simulink model "Vehicle_Model_999_Modular_roll_gradient"  (R2025b)
settings: Solver=ode23tb  StartTime=0.0  StopTime=30  MaxStep=0.001  RelTol=1e-3
values from neighbouring files (symbols this model uses):
  m = Par.m    [LapSim_Endurance_final_ts_v2.m]    (also in New_LapSim_final_ts.m = Par.Mass)
undefined symbols (not defined in the file or in its folder): Battery, Brake_Val, ctrl_Brake, ctrl_s, ctrl_Steer, ctrl_Throttle, ctrl_Velocity, HP, init_r, init_vx, init_vy, Ki_data, Kp_data, Motor, Par, steer_input, Steer_Val, sus_par, Throttle_Val, TireData, V_ref, vx_breakpoints
libraries: simulink x8, autolibshared x3, simulink_extras x2, BatteryEstimators x1
(part 3 of 3)

== matlab function Vehicle_Model_999_Modular_roll_gradient/E-powertrain/Motor/Motor with Field Weakening ==
  data: kt input; rpm_4x1 input; Torque_Nm_vec output; throttle_scalar input; v_dc_bus input; Motor parameter; I_dc_total output size=[1]; P_total_sum output size=[1]
function [Torque_Nm_vec, I_dc_total,P_total_sum] = fcn(kt, rpm_4x1, throttle_scalar, v_dc_bus, Motor)
    % Inputs:
    %   rpm_4x1         : [FL; FR; RL; RR] wheel speeds in RPM
    %   throttle_scalar : Driver input (0 to 1)
    %   v_dc_bus        : Battery voltage (V)
    %   Motor           : Struct containing constants
    
    % --- 1. Distribute Inputs ---
    % We apply the same throttle to both motors for now.
    % We extract the Rear-Left (index 3) and Rear-Right (index 4) speeds.
    rpm_targets = [rpm_4x1(3); rpm_4x1(4)]; 
    throttle_vec = [throttle_scalar; throttle_scalar];
    psi_m = kt / (1.5 * Motor.p * sqrt(2)); 

    % Initialize storage
    Torque_Nm_vec = zeros(2, 1); % [T_RL; T_RR]
    P_elec_vec = zeros(2, 1);
    
    for i = 1:2
        % --- 2. Redline & Mechanical Limit Check ---
        if abs(rpm_targets(i)) >= Motor.n_max
            continue; % Torque and Power remain 0
        end

        % --- 3. Electrical Conversions ---
        omega_m = rpm_targets(i) * (2*pi/60);
        omega_e = max(abs(omega_m * Motor.p), 0.1); 
        V_max_phase = v_dc_bus / sqrt(3);
        I_cmd_peak = Motor.I_max_rms * sqrt(2) * throttle_vec(i);

        % --- 4. Region Selection: MTPA vs Field Weakening ---
        V_req_mtpa = omega_e * sqrt((Motor.L * I_cmd_peak)^2 + psi_m^2);
        
        if V_req_mtpa <= V_max_phase
            id = 0;
            iq = I_cmd_peak;
        else
            % Field Weakening logic for Fischer Motor
            a = Motor.L^2;
            b = 2 * Motor.L * psi_m;
            c = Motor.psi_m^2 + (Motor.L * I_cmd_peak)^2 - (V_max_phase / omega_e)^2;
            
            id = (-b + sqrt(max(0, b^2 - 4 * a * c))) / (2 * a);
            id = max(min(id, 0), -I_cmd_peak); 
            iq = sqrt(max(0, I_cmd_peak^2 - id^2));
        end

        % --- 5. Torque and Power Calculation ---
        T_gen = 1.5 * Motor.p * psi_m * iq;
        Torque_Nm_vec(i) = min(T_gen, Motor.T_peak_limit);

        % P_elec = P_mechanical + P_copper_losses
        P_mech = abs(Torque_Nm_vec(i) * omega_m);
        P_copper = 3 * 0.126 * (I_cmd_peak / sqrt(2))^2;
        P_elec_vec(i) = P_mech + P_copper;
    end

    % --- 6. Battery Summation ---
    P_total_sum = sum(P_elec_vec);
    if v_dc_bus > 20
        % Calculate total current draw for the Molicel P45B pack
        I_dc_total = P_total_sum / (0.95 * v_dc_bus);

    else
        I_dc_total = 0;
    end
end

== matlab function Vehicle_Model_999_Modular_roll_gradient/Vehicle dynamics/Suspension/MATLAB Function1 ==
  data: vel input; aerodynamic_downforce output; aero_par parameter
function aerodynamic_downforce = fcn(vel,aero_par)

rho = aero_par.rho;
cd = aero_par.Cd;
A = aero_par.Area;

aerodynamic_downforce = 0.5*rho*cd*A*vel^2;

== matlab function Vehicle_Model_999_Modular_roll_gradient/Vehicle dynamics/Suspension/Roll and pitch angle calculations/Pitch_angle_calcualtions ==
  data: z_wheel input size=[4 1]; Pitch_angle output; Par parameter
function Pitch_angle = fcn(z_wheel,Par)

WB = Par.WB;

% Avg disp calculation per axle 
z_avg_f = (z_wheel(1) + z_wheel(2))/2;
z_avg_r = (z_wheel(3) + z_wheel(4))/2;

Pitch_angle = (z_avg_r- z_avg_f)/WB;

== matlab function Vehicle_Model_999_Modular_roll_gradient/Vehicle dynamics/Suspension/Roll and pitch angle calculations/Roll_angle_calulations ==
  data: z_wheel input size=[4 1]; Roll_angle output; Par parameter
function Roll_angle = fcn(z_wheel,Par)

TW = Par.TW;

% Avg disp calculation per track
z_avg_l = (z_wheel(1) + z_wheel(3))/2;
z_avg_r = (z_wheel(2) + z_wheel(4))/2;

Roll_angle = (z_avg_l - z_avg_r)/TW;

== matlab function Vehicle_Model_999_Modular_roll_gradient/Vehicle dynamics/Suspension/MATLAB Function2 ==
  data: Z_dyn input; Camber output; Camber_gain output; HP parameter; sus_par parameter
function [Camber, Camber_gain] = DynamicCamber_FromHP_Zmeters(Z_dyn, HP, sus_par)
%#codegen
% Z_dyn : dynamic wheel vertical displacement from static ride height (meters, + = bump)
% Output Camber [4x1] radians (dynamic absolute camber)

% 1. Configured static camber
static_camber_4x1 = sus_par.Camber_static .* ones(4,1);

% 2. Dynamic displacements in mm (FL, FR, RL, RR)
zw = Z_dyn .* [sus_par.Motion_ratio_f; sus_par.Motion_ratio_f; ...
               sus_par.Motion_ratio_r; sus_par.Motion_ratio_r] .* 1000;

% 3. Extract and Vectorize Hardpoints (Applying side mirroring directly)
% Inner Pivots (Y and Z) - Average of F and R legs to establish the inner pivot axis
UiY = [ (HP.Front.UCA_F(2) + HP.Front.UCA_R(2))*0.5;
       -(HP.Front.UCA_F(2) + HP.Front.UCA_R(2))*0.5;
        (HP.Rear.UCA_F(2)  + HP.Rear.UCA_R(2))*0.5;
       -(HP.Rear.UCA_F(2)  + HP.Rear.UCA_R(2))*0.5 ];

UiZ = [ (HP.Front.UCA_F(3) + HP.Front.UCA_R(3))*0.5;
        (HP.Front.UCA_F(3) + HP.Front.UCA_R(3))*0.5;
        (HP.Rear.UCA_F(3)  + HP.Rear.UCA_R(3))*0.5;
        (HP.Rear.UCA_F(3)  + HP.Rear.UCA_R(3))*0.5 ];

LiY = [ (HP.Front.LCA_F(2) + HP.Front.LCA_R(2))*0.5;
       -(HP.Front.LCA_F(2) + HP.Front.LCA_R(2))*0.5;
        (HP.Rear.LCA_F(2)  + HP.Rear.LCA_R(2))*0.5;
       -(HP.Rear.LCA_F(2)  + HP.Rear.LCA_R(2))*0.5 ];

LiZ = [ (HP.Front.LCA_F(3) + HP.Front.LCA_R(3))*0.5;
        (HP.Front.LCA_F(3) + HP.Front.LCA_R(3))*0.5;
        (HP.Rear.LCA_F(3)  + HP.Rear.LCA_R(3))*0.5;
        (HP.Rear.LCA_F(3)  + HP.Rear.LCA_R(3))*0.5 ];

% Outer Pivots (Y and Z base static values)
UO_Y = [HP.Front.UCA_O(2); -HP.Front.UCA_O(2); HP.Rear.UCA_O(2); -HP.Rear.UCA_O(2)];
LO_Y = [HP.Front.LCA_O(2); -HP.Front.LCA_O(2); HP.Rear.LCA_O(2); -HP.Rear.LCA_O(2)];
TCP_Y = [HP.Front.TCP(2);  -HP.Front.TCP(2);  HP.Rear.TCP(2);  -HP.Rear.TCP(2)];

UO_Z_base  = [HP.Front.UCA_O(3); HP.Front.UCA_O(3); HP.Rear.UCA_O(3); HP.Rear.UCA_O(3)];
LO_Z_base  = [HP.Front.LCA_O(3); HP.Front.LCA_O(3); HP.Rear.LCA_O(3); HP.Rear.LCA_O(3)];
TCP_Z_base = [HP.Front.TCP(3);   HP.Front.TCP(3);   HP.Rear.TCP(3);   HP.Rear.TCP(3)];

% 4. Compute Kinematics Vectorized (All 4 corners at once)
% Dynamic geometry
Camber_d = compute_corner_kinematics(zw, UiY, UiZ, LiY, LiZ, UO_Y, LO_Y, TCP_Y, UO_Z_base, LO_Z_base, TCP_Z_base);

% Static geometry (0 mm travel)
Camber_s_raw = compute_corner_kinematics([0;0;0;0], UiY, UiZ, LiY, LiZ, UO_Y, LO_Y, TCP_Y, UO_Z_base, LO_Z_base, TCP_Z_base);
Camber_s = abs(Camber_s_raw); % Mirroring your original solveCorner_theta logic

% 5. Calculate Deltas (Preserving your exact original quadrant/sign logic)
Camber_delta = [
    -Camber_s(1) + Camber_d(1);
    -Camber_d(2) - Camber_s(2);
     Camber_d(3) - Camber_s(3);
    -Camber_d(4) - Camber_s(4)
];

% 6. Final Outputs
Camber = Camber_delta + static_camber_4x1;
Camber_gain = Camber_d;
static_camber_visualisation = Camber_s;

end

%% High-Performance Vectorized Helper Function
function Camber_rad = compute_corner_kinematics(zw, UiY, UiZ, LiY, LiZ, UO_Y, LO_Y, TCP_Y, UO_Z_base, LO_Z_base, TCP_Z_base)
    % Apply vertical travel
    UO_Z  = UO_Z_base + zw;
    LO_Z  = LO_Z_base + zw;
    TCP_Z = TCP_Z_base + zw;

    % Slopes of upper & lower arms
    dYU = UO_Y - UiY;
    dYL = LO_Y - LiY;

    % Singularity protection (Replaces previous 0*sign(0) bug)
    dYU = protect_zero(dYU, 1e-6);
    dYL = protect_zero(dYL, 1e-6);

    mU = (UO_Z - UiZ) ./ dYU;
    mL = (LO_Z - LiZ) ./ dYL;

    cU = UiZ - mU .* UiY;
    cL = LiZ - mL .* LiY;

    % Instant Center (IC) Calculation
    den = mU - mL;
    den = protect_zero(den, 1e-6);

    ICy = (cL - cU) ./ den;
    ICz = mU .* ICy + cU;

    % Camber from IC to Contact Patch
    dY = ICy - TCP_Y;
    dZ = ICz - TCP_Z;
    dZ = protect_zero(dZ, 1e-6);

    Camber_rad = -atan(dY ./ dZ);
end

%% Singularity Protection Helper (Coder Safe)
function out = protect_zero(val, tol)
    out = val;
    for i = 1:4
        if abs(out(i)) < tol
            s = sign(out(i));
            if s == 0
                s = 1;
            end
            out(i) = s * tol;
        end
    end
end

== matlab function Vehicle_Model_999_Modular_roll_gradient/Vehicle dynamics/Fx, Fy calculations/Tyre_relaxation/MATLAB Function ==
  data: Fx_ss input; Fx_dot output; Fx_act input; Vx input
function Fx_dot = fcn(Fx_ss, Fx_act, Vx)
    % Fx_ss: Force from Magic Formula block
    % Fx_act: The current integrated force
    % Vx: Longitudinal velocity
    sigma_x = 0.1;
    % Use a small epsilon to avoid division by zero at standstill
    Vx_mod = max(abs(Vx), 0.05); 
    
    % The differential equation
    Fx_dot = (Vx_mod / sigma_x).* (Fx_ss - Fx_act);
end

== matlab function Vehicle_Model_999_Modular_roll_gradient/Vehicle dynamics/Fx, Fy calculations/Visualise_Fy_B/MATLAB Function ==
  data: Fy_tire input; Fy_B_fl output; Fy_B_fr output; Fy_B_rl output; Fy_B_rr output
function [Fy_B_fl,Fy_B_fr,Fy_B_rl,Fy_B_rr]  = fcn(Fy_tire)

Fy_B_fl = Fy_tire(1);

Fy_B_fr = Fy_tire(2);

Fy_B_rl = Fy_tire(3);

Fy_B_rr = Fy_tire(4);

end

== matlab function Vehicle_Model_999_Modular_roll_gradient/Drivetrain/MATLAB Function ==
  data: T_fl output; T_fr output
function [T_fl,T_fr] = fcn()

T_fl = 0;
T_fr = 0;

== matlab function Vehicle_Model_999_Modular_roll_gradient/E-powertrain/Motor/rpm selection for third wheel ==
  data: u input; y output
function y = fcn(u)

y = u(3);

== matlab function Vehicle_Model_999_Modular_roll_gradient/Vehicle dynamics/Fx, Fy calculations/Slip_angle_calculation/Slip Angles ==
  data: Longitudinal_vel input; slip_angles output; Lateral_vel input; yawrate input; Steer_FL input; Steer_FR input; Par parameter
function slip_angles = fcn(Longitudinal_vel, Lateral_vel, yawrate, Steer_FL, Steer_FR, Par)
%#codegen

    % 1. Geometry Setup
    L = Par.WB;
    T = Par.TW;
    
    % Distance from CG to Axles
    a = L * Par.WD_r;     
    b = L - a;             
    half_T = T / 2;

    % 2. Calculate Velocity Components at Each Corner
    % Kinematic transformation from CG to Hubs
    % Front Left (1)
        Vx_FL = Longitudinal_vel - yawrate * half_T;
        Vy_FL = Lateral_vel + yawrate * a;
    
    % Front Right (2)
        Vx_FR = Longitudinal_vel + yawrate * half_T;
        Vy_FR = Lateral_vel + yawrate * a;
    
    % Rear Left (3)
        Vx_RL = Longitudinal_vel - yawrate * half_T;
        Vy_RL = Lateral_vel - yawrate * b;
    
    % Rear Right (4)
        Vx_RR = Longitudinal_vel + yawrate * half_T;
        Vy_RR = Lateral_vel - yawrate * b;

    % 3. Calculate Velocity Angles (Theta_V)

        Theta_FL = atan2(Vy_FL, max(Vx_FL,0.001)); 
        Theta_FR = atan2(Vy_FR, max(Vx_FR,0.001));
        Theta_RL = atan2(Vy_RL, max(Vx_RL,0.001));
        Theta_RR = atan2(Vy_RR, max(Vx_RR,0.001));
    
    % 4. Construct Steering Vector (Delta)
    % Rears are assumed fixed (0 steering)
        Delta = [Steer_FL; Steer_FR; 0; 0];
    
    % Vector of Velocity Angles
        Theta_V = [Theta_FL; Theta_FR; Theta_RL; Theta_RR];

    % 5. Final Calculation
    % Alpha = Delta - Theta_V
        slip_angles = Delta - Theta_V ;
end

== matlab function Vehicle_Model_999_Modular_roll_gradient/Vehicle dynamics/Fx, Fy calculations/Slip_ratio_calculation/slip ratios ==
  data: Vx input; Vy input; slip_ratios output; yawrate input; Omega input; Steer_FL input; Steer_FR input; Par parameter
function slip_ratios = fcn(Vx,Vy, yawrate, Omega,Steer_FL,Steer_FR, Par)
%#codegen


    % 1. Constants
    T = Par.TW;
    Re = Par.R0;
    half_T = T / 2;
    a= Par.Lf;
    b=Par.Lr;
    r = yawrate;
    % 2 Yaw Rate Correction (Kinematics)
    
    Vx_FL = Vx - yawrate * half_T;  % Left
    Vx_FR = Vx + yawrate * half_T;  % Right
    Vx_RL = Vx - yawrate * half_T;
    Vx_RR = Vx + yawrate * half_T;
    
    Vx_vec = [Vx_FL; Vx_FR; Vx_RL; Vx_RR];
    
    Vy_FL = Vy + r * a;
    Vy_FR = Vy+ r * a;
    Vy_RL = Vy- r * b;
    Vy_RR = Vy- r * b;

    Vy_vec = [Vy_FL; Vy_FR; Vy_RL; Vy_RR];
    Delta = [Steer_FL;Steer_FR;0;0];
    % 3. Slip Angle Correction (Projection)
 
    V_road_plane = Vx_vec .* cos(Delta) + Vy_vec .* sin(Delta);

    % 4. Calculate Wheel Linear Speed
    V_wheel = Omega .* Re;

    % 5. Calculate Slip Ratio
    V_safe_threshold = 0.1; 
    V_ref = max(abs(V_road_plane), V_safe_threshold);
    
    slip_ratios_raw = (V_wheel - V_road_plane) ./ V_ref;
    slip_ratios = slip_ratios_raw;
    % slip_ratios = min(max(slip_ratios_raw,-1),1);
end

== matlab function Vehicle_Model_999_Modular_roll_gradient/Vehicle dynamics/Steering/Steering Kinematics/Steering Kinematics ==
  data: Steer_Input input; Ackermann_Pct input; Steer_FL output; Steer_FR output; Par parameter
function [Steer_FL, Steer_FR] = fcn(Steer_Input, Ackermann_Pct, Par)
%#codegen

    % 1. Constants
    L = Par.WB;      % Wheelbase
    half_T = Par.TW / 2; % Half Track Width

    % 2. Safety Clamp (Prevent tan(90) singularity)
    delta = min(max(Steer_Input, -1.5), 1.5); 
    
    % 3. Calculate "Pure Ackermann" Angles
    % Ideally, inner wheel turns sharper than outer wheel.
    tan_d = tan(delta);
    
    % FL (Left): Denom depends on sign of turn.
    % If turning Left (+), Denom shrinks (Sharper).
    FL_Ack = atan( (L * tan_d) / (L - half_T * tan_d) );
    
    % FR (Right): 
    % If turning Left (+), Denom grows (Shallower).
    FR_Ack = atan( (L * tan_d) / (L + half_T * tan_d) );
    
    % 4. Calculate "Parallel" Angles
    % Both wheels exactly match the center input
    FL_Par = delta;
    FR_Par = delta;
    
    % 5. Linear Blend based on Percentage
    % Formula: Final = Parallel + (Ackermann - Parallel) * Percent
    Steer_FL = FL_Par + (FL_Ack - FL_Par) * Ackermann_Pct;
    Steer_FR = FR_Par + (FR_Ack - FR_Par) * Ackermann_Pct;

end

== matlab function Vehicle_Model_999_Modular_roll_gradient/Vehicle dynamics/Fx, Fy calculations/Simplified Tire Model ==
  data: Fz input; Fx output size=4; slip_ratios input; slip_angles input; camber_angles input; Fy output size=4; Self_aligning_torque output size=4; Mu_x output size=4; Mu_y output size=4; TireData parameter; Par parameter; sus_par parameter; Dy output size=[4 1]
function [Fx, Fy, Self_aligning_torque, Mu_x, Mu_y, Dy] = fcn(Fz, slip_ratios, slip_angles, camber_angles, TireData, Par, sus_par)
%#codegen
% =========================================================================
%  VECTORIZED MAGIC FORMULA 5.2 (4-WHEEL)
% =========================================================================

    % 0. Enforce Column Vectors (Crash Protection)
    Fz = Fz(:);
    slip_ratios = slip_ratios(:);
    slip_angles = slip_angles(:);
    camber_angles = camber_angles(:);

    % 1. EXTRACT PARAMETERS (Scalars)
    p = TireData;
    s = TireData.Scales;
    Fz0 = p.FNOMIN;
    R0  = p.R0;
    par = Par;
    
    % 2. INPUT SAFETY & NORMALIZATION
    % Clamp negative loads to 0 (Tires can't pull ground)
    Fz_safe = max(Fz, 0); 
    
    % Avoid division by zero for Mu calculations later
    Fz_denom = max(Fz_safe, 1.0); 
    
    % Normalized Load (dfz) - Vectorized
    dfz = (Fz_safe - Fz0) ./ Fz0;
    
    % ---------------------------------------------------------------------
    % A. LONGITUDINAL FORCE (Fx) - VECTORIZED
    % ---------------------------------------------------------------------
    Cx = p.PCX1 * s.LCX;
    
    % Friction Coeff Mu_x
    mu_x_base = (p.PDX1 + p.PDX2 .* dfz) .* (1 - p.PDX3 .* camber_angles.^2) .* s.LMUX;
    Dx = mu_x_base .* Fz_safe;
    
    % Stiffness Kx
    Kx = Fz_safe .* (p.PKX1 + p.PKX2 .* dfz) .* exp(p.PKX3 .* dfz) .* s.LKX;
    
    % Stiffness Factor Bx
    Bx = Kx ./ (Cx .* Dx + 1e-6); 
    
    % Shifts (Horizontal & Vertical)
    Shx = (p.PHX1 + p.PHX2 .* dfz) .* s.LHX;
    Svx = Fz_safe .* (p.PVX1 + p.PVX2 .* dfz) .* s.LVX;
    
    % Composite Slip
    k_s = slip_ratios + Shx;
    
    % Curvature Ex (Sign Dependent)
    Ex = (p.PEX1 + p.PEX2 .* dfz + p.PEX3 .* dfz.^2) .* (1 - p.PEX4 .* sign(k_s)) .* s.LEX;
    Ex(Ex > 1) = 1; % Clamp
    
    % Calculation
    Bx_k = Bx .* k_s;
    Fx = Dx .* sin(Cx .* atan(Bx_k - Ex .* (Bx_k - atan(Bx_k)))) + Svx;
    
    % ---------------------------------------------------------------------
    % B. LATERAL FORCE (Fy) - VECTORIZED
    % ---------------------------------------------------------------------
    Cy = p.PCY1 * s.LCY;
    
    % Friction Coeff Mu_y
    mu_y_base = (p.PDY1 + p.PDY2 .* dfz) .* (1 - p.PDY3 .* camber_angles.^2) .* s.LMUY;
    Dy = mu_y_base .* Fz_safe;
    
    % Cornering Stiffness Ky (Trig Form)
    Ky = p.PKY1 .* Fz0 .* sin(2 .* atan(Fz_safe ./ (p.PKY2 .* Fz0))) .* (1 - p.PKY3 .* abs(camber_angles)) .* s.LKY;
    
    % Poly fallback check (if PKY2 implies poly form)
    if (Ky(1) < 1)
        Ky = Fz_safe .* (p.PKY1 + p.PKY2 .* dfz) .* s.LKY;
    end
    
    By = Ky ./ (Cy .* Dy + 1e-6);
    
    % Shifts 
    Shy = (p.PHY1 + p.PHY2 .* dfz) .* s.LHY;
    Svy = Fz_safe .* (p.PVY1 + p.PVY2 .* dfz) .* s.LVY;
    
    % FIXED: Removed the 0* debug multiplier
    a_s = slip_angles + Shy;
    
    % Curvature Ey (Sign Dependent)
    Ey = (p.PEY1 + p.PEY2 .* dfz) .* (1 - (p.PEY3 + p.PEY4 .* camber_angles) .* sign(a_s)) .* s.LEY;
    Ey(Ey > 1) = 1;
    
    % Calculation
    By_a = By .* a_s;
    % FIXED: Removed the 0* debug multiplier
    Fy = -(Dy .* sin(Cy .* atan(By_a - Ey .* (By_a - atan(By_a)))) + Svy);
    
    % ---------------------------------------------------------------------
    % C. SELF-ALIGNING TORQUE (Mz) - VECTORIZED
    % ---------------------------------------------------------------------
    % Peak Trail Dt
    Dt = (p.QDZ1 + p.QDZ2 .* dfz) .* (1 - p.QDZ3 .* abs(camber_angles)) .* R0 .* s.LTR;
    
    % Trail Slope Bt
    Bt = (p.QBZ1 + p.QBZ2 .* dfz + p.QBZ3 .* dfz.^2) .* (1 + p.QBZ4 .* abs(camber_angles)) .* (s.LKY / s.LMUY);
    
    Ct = p.QCZ1; % Scalar
    Et = (p.QEZ1 + p.QEZ2 .* dfz + p.QEZ3 .* dfz.^2);
    
    % Trail 't' Calculation(Pneumatic trail)
    Bt_a = Bt .* a_s;
    alpha_t = Bt_a - Et .* (Bt_a - atan(Bt_a));
    t = Dt .* cos(Ct .* atan(alpha_t)) .* cos(a_s);
    
    % Trail 'tm' Calculation(mechanical trail)
    tm = par.R0 .* tan(sus_par.Caster_static);
    
    % Residual Mzr
    Dr = Fz_safe .* R0 .* (p.QDZ6 + p.QDZ7 .* dfz) .* s.LRES;
    Br = 10;
    Mzr = Dr .* cos(atan(Br .* a_s));
    
    % Final Mz (Standard Restoring: Negative Slope)
    Self_aligning_torque = -(t + tm) .* Fy + Mzr;
    
    % ---------------------------------------------------------------------
    % D. OUTPUTS 
    % ---------------------------------------------------------------------
    % Friction Coeffs
    Mu_x = Fx ./ Fz_denom;
    Mu_y = Fy ./ Fz_denom;
    
    % Note on Lifted Wheels: Because Fz_safe mathematically zeroes out 
    % Dx, Kx, Dy, Ky, Dt, and Dr, the outputs smoothly evaluate to 0 
    % without needing the commented-out boolean masking. 
    % This is faster and safer for C-code generation.
end
